simulink model "tema2_mdl"  (R2019a)
settings: Solver=VariableStepAuto  StartTime=0.0  StopTime=400  RelTol=1e-3
values from neighbouring files (symbols this model uses):
  r = 2 * ystar    [tema2.m]
  sys = ss(S.a, S.b, S.c, S.d)    [tema2.m]
  ustar = zeros(10,1)    [tema1.m]
undefined symbols (not defined in the file or in its folder): xstar, ystar
settings Model: Creator=cynthia  LastModifiedBy=cynthia

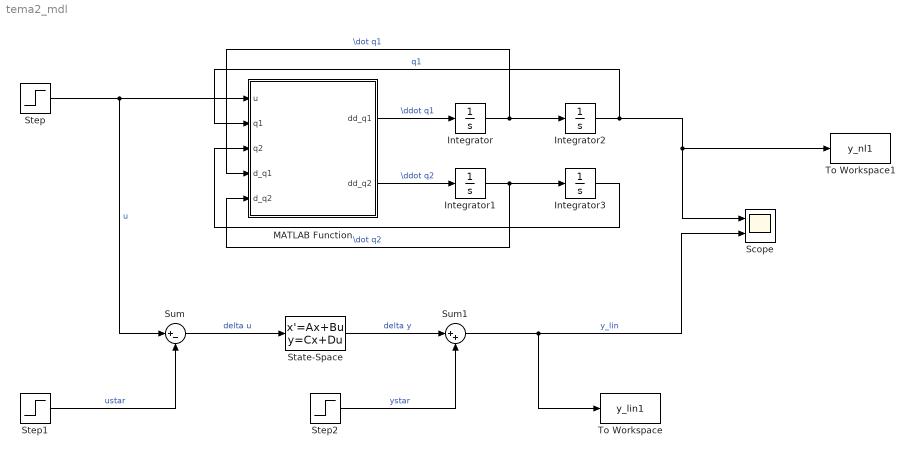
== system tema2_mdl ==
  Integrator{,1..3} (4 alike) : Integrator
  MATLAB Function : MATLAB Function  TreatAsAtomicUnit=on
  Scope : Scope  NumInputPorts=2
  State-Space : StateSpace  A=sys.A  B=sys.B  C=sys.C  D=sys.D  InitialCondition=[0;0;0;0] - xstar
  Step : Step  Time=0  After=r  SampleTime=0
  Step1 : Step  Time=0  After=ustar  SampleTime=0
  Step2 : Step  Time=0  After=ystar  SampleTime=0
  Sum : Sum  Inputs=|+-
  Sum1 : Sum  Inputs=|++
  To Workspace : ToWorkspace  VariableName=y_lin1  SaveFormat=Timeseries  SampleTime=-1
  To Workspace1 : ToWorkspace  VariableName=y_nl1  SaveFormat=Timeseries  SampleTime=-1
  wires:
  MATLAB Function/1(dd_q1) -> Integrator/1  "\\ddot q1"
  Integrator/1 -> Integrator2/1, MATLAB Function/4(d_q1)  "\\dot q1"
  MATLAB Function/2(dd_q2) -> Integrator1/1  "\\ddot q2"
  Integrator1/1 -> Integrator3/1, MATLAB Function/5(d_q2)  "\\dot q2"
  Step/1 -> Sum/1, MATLAB Function/1(u)  "u"
  Integrator2/1 -> To Workspace1/1, Scope/1, MATLAB Function/2(q1)  "q1"
  Integrator3/1 -> MATLAB Function/3(q2)
  State-Space/1 -> Sum1/1  "delta y"
  Sum/1 -> State-Space/1  "delta u"
  Step1/1 -> Sum/2  "ustar"
  Step2/1 -> Sum1/2  "ystar"
  Sum1/1 -> To Workspace/1, Scope/2  "y_lin"

== matlab function tema2_mdl/MATLAB Function ==
  data: u input; dd_q1 output; q1 input; q2 input; d_q1 input; d_q2 input; dd_q2 output
function [dd_q1,dd_q2] = fcn(u,q1,q2,d_q1,d_q2)
m = 5.1;
g = 10;
L = 1.56;
zeta = 7.64;
k = 0.25;
J = 2.77; 
I = 1.89;
M = 2.82;

dd_q1 = (u + k*(q2-q1) - zeta*d_q1)/J;
dd_q2 = (-M*g*L*sin(q2) - k*(q2-q1) - zeta*d_q2)/I;


end
